simulink model "System_Model"  (Simulink 7.6)
settings: Solver=ode15s  StartTime=0.0  StopTime=50  RelTol=1e-3
undefined symbols (not defined in the file): C, DiscIntNeverNeededParam, F, G, g, H, K, L0, m, magnitude, Nu, Nx, Q, R, u0, x01, x02, x03
libraries: fl_lib x18, nesl_utility x5, simulink x3, elec_lib x1
CloseFcn:
  | rtwprivate ssgencode ModelCloseRequest System_Model1
settings Model: Creator=Fodi  LastModifiedBy=Fodi

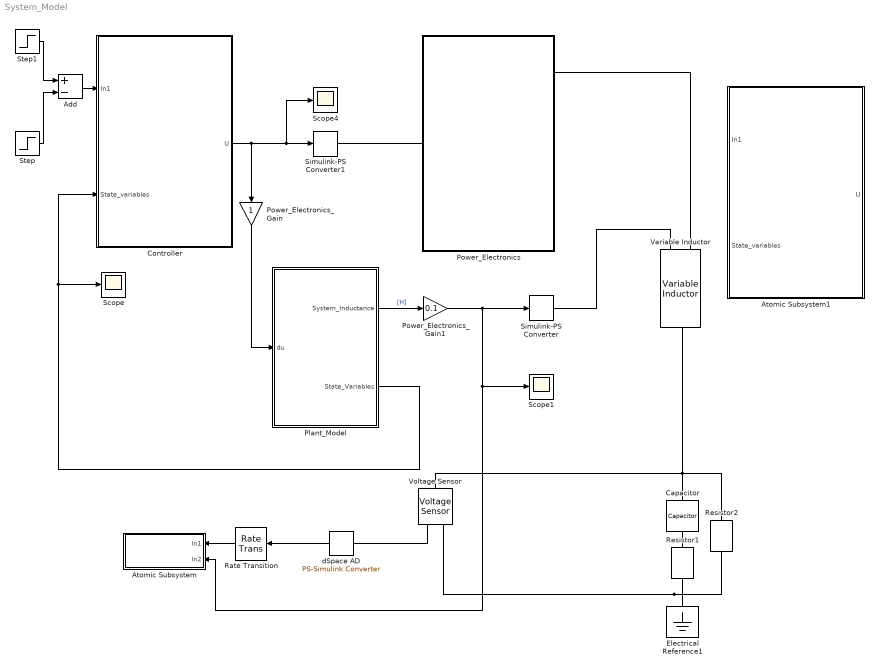
== system System_Model ==
  Add : Sum  Inputs=+-
  Atomic Subsystem : Subsystem  TreatAsAtomicUnit=on
  Atomic Subsystem1 : Subsystem  TreatAsAtomicUnit=on
  Capacitor : fl_lib/Electrical/Electrical Elements/Capacitor  DialogController=NetworkEngine.DynNeDlgSource  SystemSampleTime=-1  c=1e-6 F  v0=0 V  r=1e-6 Ohm  g=0 1/Ohm  i_Log=off  v_Log=off  vc_Log=off  LocalVarNames=|i|v|vc  LocalVarDescs=|i|v|Internal variable for voltage across capacitor term  LocalVarLogging=[0 0 0]
  Controller : Subsystem
  Electrical Reference1 : fl_lib/Electrical/Electrical Elements/Electrical Reference  DialogController=NetworkEngine.DynNeDlgSource  SystemSampleTime=-1  i_Log=off  LocalVarNames=|i  LocalVarDescs=|i  LocalVarLogging=0
  Plant_Model : Subsystem
  Power_Electronics : Subsystem
  Power_Electronics_Gain : Gain
  Power_Electronics_Gain1 : Gain  Gain=0.1
  Rate Transition : RateTransition  OutPortSampleTime=0.001
  Resistor1 : fl_lib/Electrical/Electrical Elements/Resistor  DialogController=NetworkEngine.DynNeDlgSource  SystemSampleTime=-1  R=17 Ohm  i_Log=off  v_Log=off  LocalVarNames=|i|v  LocalVarDescs=|i|v  LocalVarLogging=[0 0]
  Resistor2 : fl_lib/Electrical/Electrical Elements/Resistor  DialogController=NetworkEngine.DynNeDlgSource  SystemSampleTime=-1  R=17 Ohm  i_Log=off  v_Log=off  LocalVarNames=|i|v  LocalVarDescs=|i|v  LocalVarLogging=[0 0]
  Scope : Scope
      settings: YMin=0.00025  YMax=0.00575  SaveName=ScopeData7
  Scope1 : Scope
      settings: YMin=0.266286  YMax=0.266289  SaveName=ScopeData5
  Scope4 : Scope
      settings: YMin=0.1375  YMax=0.142  SaveName=ScopeData6
  Simulink-PS Converter : nesl_utility/Simulink-PS Converter  DialogController=NetworkEngine.DynNeUtilDlgSource  SystemSampleTime=-1  PhysicalDomain=network_engine_domain  LeftPortType=input  RightPortType=output  SubClassName=ps_input  Unit=1  AffineConversion=off  InputFilterTimeConstant=.001  UdotUserProvided=0
  Simulink-PS Converter1 : nesl_utility/Simulink-PS Converter  DialogController=NetworkEngine.DynNeUtilDlgSource  SystemSampleTime=-1  PhysicalDomain=network_engine_domain  LeftPortType=input  RightPortType=output  SubClassName=ps_input  Unit=1  AffineConversion=off  InputFilterTimeConstant=.001  UdotUserProvided=0
  Step : Step  Time=20  After=0.0003  SampleTime=0
  Step1 : Step  Time=0  After=0.001  SampleTime=0
  Variable Inductor : elec_lib/Passive Devices/Variable Inductor  DialogController=NetworkEngine.DynNeDlgSource  SystemSampleTime=-1  prm=2  Lmin=1e-6 H  g=1e-9 1/Ohm  i0=0 A  phi0=0 Wb  LocalVarLogging=[]
  Voltage Sensor : fl_lib/Electrical/Electrical Sensors/Voltage Sensor  DialogController=NetworkEngine.DynNeDlgSource  SystemSampleTime=-1  i1_Log=off  v1_Log=off  LocalVarNames=|i1|v1  LocalVarDescs=|i1|v1  LocalVarLogging=[0 0]
  dSpace AD : nesl_utility/PS-Simulink Converter  DialogController=NetworkEngine.DynNeUtilDlgSource  SystemSampleTime=-1  PhysicalDomain=network_engine_domain  LeftPortType=input  RightPortType=output  SubClassName=ps_output  Unit=1  AffineConversion=off
  wires:
  Plant_Model/1(System_Inductance) -> Power_Electronics_Gain1/1  "[H]"
  Controller/1(U) -> Power_Electronics_Gain/1, Simulink-PS Converter1/1, Scope4/1
  Power_Electronics_Gain/1 -> Plant_Model/1(du)
  Plant_Model/2(State_Variables) -> Controller/2(State_variables), Scope/1
  Power_Electronics_Gain1/1 -> Simulink-PS Converter/1, Atomic Subsystem/2(In2), Scope1/1
  Add/1 -> Controller/1(In1)
  Step1/1 -> Add/1
  Step/1 -> Add/2
  dSpace AD/1 -> Rate Transition/1
  Rate Transition/1 -> Atomic Subsystem/1(In1)
  connections:
  Simulink-PS Converter1/RConn1 -- Power_Electronics/LConn1
  Power_Electronics/RConn1 -- Variable Inductor/LConn2
  Variable Inductor/RConn1 -- Voltage Sensor/LConn1 -- Capacitor/LConn1 -- Resistor2/LConn1
  Resistor1/RConn1 -- Electrical Reference1/LConn1 -- Voltage Sensor/RConn2 -- Resistor2/RConn1
  Simulink-PS Converter/RConn1 -- Variable Inductor/LConn1
  Voltage Sensor/RConn1 -- dSpace AD/LConn1
  Capacitor/RConn1 -- Resistor1/LConn1

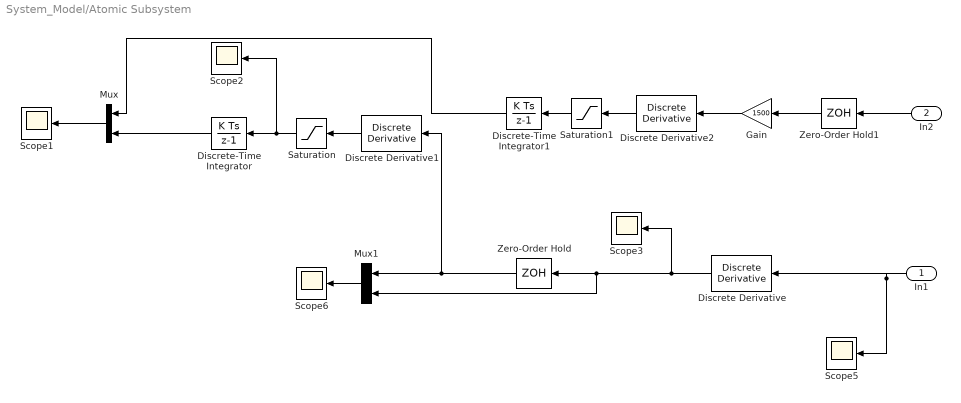
== system System_Model/Atomic Subsystem ==
  In1 : Inport
  In2 : Inport  Port=2
  Discrete Derivative : simulink/Discrete/Discrete Derivative  SystemSampleTime=-1  gainval=1.0  ICPrevScaledInput=0.0  OutMin=[]  OutMax=[]  OutDataType=fixdt(1, 16)  OutScaling=2^-10  DoSatur=off
  Discrete Derivative1 : simulink/Discrete/Discrete Derivative  SystemSampleTime=-1  gainval=1.0  ICPrevScaledInput=0.0  OutMin=[]  OutMax=[]  OutDataType=fixdt(1, 16)  OutScaling=2^-10  DoSatur=off
  Discrete Derivative2 : simulink/Discrete/Discrete Derivative  SystemSampleTime=-1  gainval=1.0  ICPrevScaledInput=0.0  OutMin=[]  OutMax=[]  OutDataType=fixdt(1, 16)  OutScaling=2^-10  DoSatur=off
  Discrete-Time Integrator : DiscreteIntegrator  SampleTime=-1  ICPrevOutput=DiscIntNeverNeededParam  ICPrevScaledInput=DiscIntNeverNeededParam
  Discrete-Time Integrator1 : DiscreteIntegrator  SampleTime=-1  ICPrevOutput=DiscIntNeverNeededParam  ICPrevScaledInput=DiscIntNeverNeededParam
  Gain : Gain  Gain=1500
  Mux : Mux  Inputs=2
  Mux1 : Mux  Inputs=2
  Saturation : Saturate  UpperLimit=10  LowerLimit=-10
  Saturation1 : Saturate  UpperLimit=10  LowerLimit=-10
  Scope{1..3,5..6} (5 alike) : Scope
      Scope1 settings: YMin=-6  YMax=-1.75  SaveName=ScopeData9
      Scope2 settings: YMin=-1.75e-008  YMax=2e-008  SaveName=ScopeData10
      Scope3 settings: YMin=-600  YMax=600  SaveName=ScopeData8
      Scope5 settings: YMin=-0.43  YMax=-0.2  SaveName=ScopeData11
      Scope6 settings: YMin=18.8348  YMax=18.8348  SaveName=ScopeData16
  Zero-Order Hold : ZeroOrderHold  SampleTime=1/20
  Zero-Order Hold1 : ZeroOrderHold  SampleTime=1/20
  wires:
  In1/1 -> Scope5/1, Discrete Derivative/1
  Zero-Order Hold/1 -> Discrete Derivative1/1, Mux1/1
  Discrete Derivative/1 -> Scope3/1, Zero-Order Hold/1, Mux1/2
  Saturation/1 -> Discrete-Time Integrator/1, Scope2/1
  Mux/1 -> Scope1/1
  Discrete-Time Integrator/1 -> Mux/2
  In2/1 -> Zero-Order Hold1/1
  Gain/1 -> Discrete Derivative2/1
  Discrete Derivative2/1 -> Saturation1/1
  Saturation1/1 -> Discrete-Time Integrator1/1
  Discrete-Time Integrator1/1 -> Mux/1
  Zero-Order Hold1/1 -> Gain/1
  Discrete Derivative1/1 -> Saturation/1
  Mux1/1 -> Scope6/1

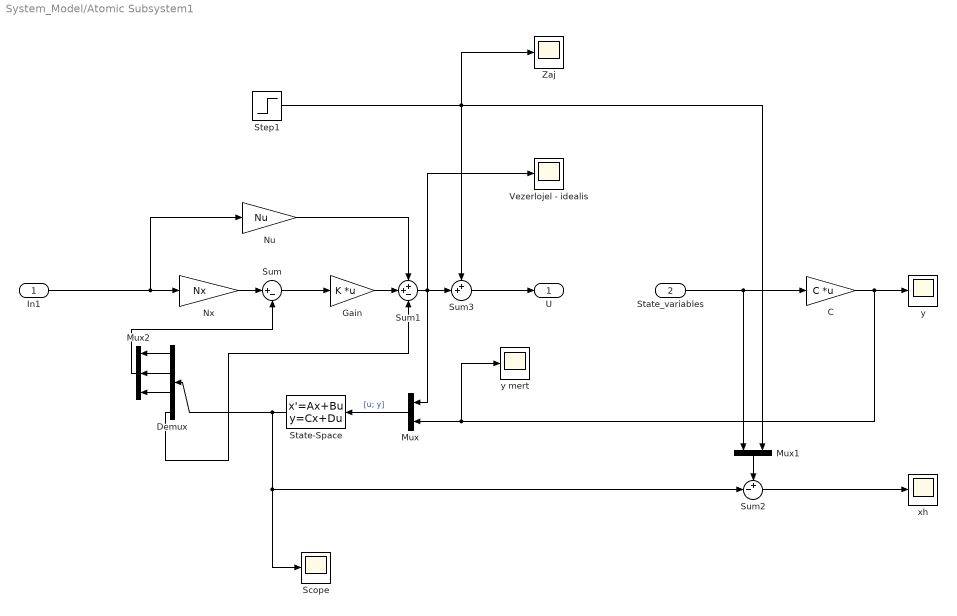
== system System_Model/Atomic Subsystem1 ==
  In1 : Inport
  State_variables : Inport  Port=2
  C : Gain  Gain=C  Multiplication=Matrix(K*u)
  Demux : Demux
  Gain : Gain  Gain=K  Multiplication=Matrix(K*u)
  Mux : Mux  Inputs=2
  Mux1 : Mux  Inputs=2
  Mux2 : Mux  Inputs=3
  Nu : Gain  Gain=Nu
  Nx : Gain  Gain=Nx
  Scope : Scope
      settings: SaveName=xb1
  State-Space : StateSpace  A=F  B=[H G]  C=eye(size(F))  D=zeros(size(F,1),size([H G],2))
  Step1 : Step  Time=2  After=0  SampleTime=0
  Sum : Sum  Inputs=|+-
  Sum1 : Sum  Inputs=++-
  Sum2 : Sum  Inputs=+-|
  Sum3 : Sum  Inputs=++|
  Vezerlojel - idealis : Scope
      settings: TimeRange=10  YMin=-1  YMax=3  SaveName=u1
  Zaj : Scope
      settings: SaveName=ScopeData12
  xh : Scope
      settings: TimeRange=10  YMin=-0.02  YMax=0.12  SaveName=ScopeData13
  y : Scope
      settings: TimeRange=10  YMin=0  YMax=0.0025  SaveName=y1
  y mert : Scope
      settings: TimeRange=5  YMin=0  YMax=0.003  SaveName=ym1
  U : Outport
  wires:
  In1/1 -> Nx/1, Nu/1
  Nx/1 -> Sum/1
  Nu/1 -> Sum1/1
  Gain/1 -> Sum1/2
  Sum/1 -> Gain/1
  Sum1/1 -> Mux/1, Sum3/2, Vezerlojel - idealis/1
  State_variables/1 -> C/1, Mux1/1
  State-Space/1 -> Demux/1, Sum2/2, Scope/1
  Mux/1 -> State-Space/1  "[u; y]"
  Step1/1 -> Sum3/1, Mux1/2, Zaj/1
  Sum3/1 -> U/1
  Mux1/1 -> Sum2/1
  Mux2/1 -> Sum/2
  Demux/4 -> Sum1/3
  Demux/1 -> Mux2/1
  Demux/2 -> Mux2/2
  Demux/3 -> Mux2/3
  Sum2/1 -> xh/1
  C/1 -> y/1, Mux/2, y mert/1

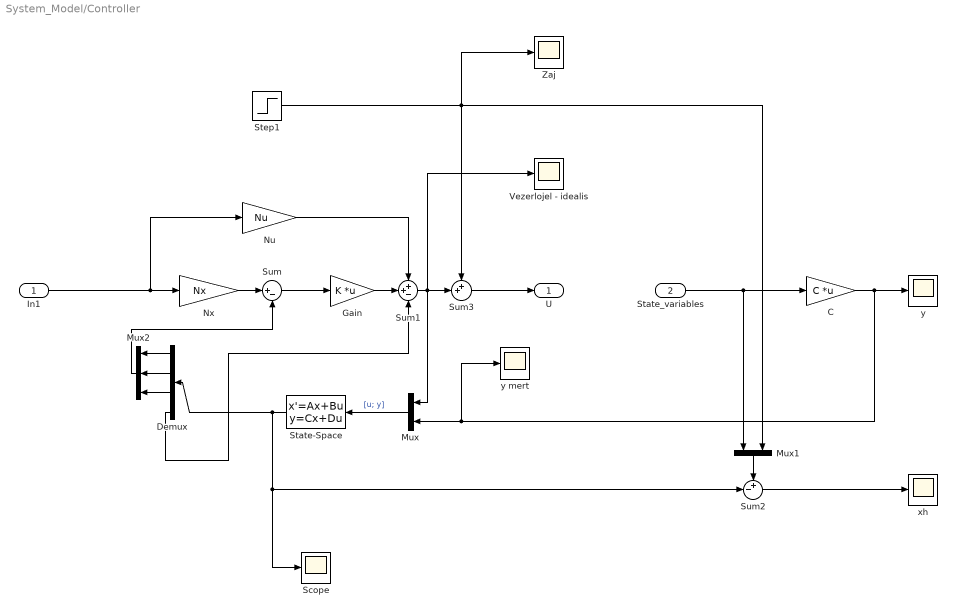
== system System_Model/Controller ==
  In1 : Inport
  State_variables : Inport  Port=2
  C : Gain  Gain=C  Multiplication=Matrix(K*u)
  Demux : Demux
  Gain : Gain  Gain=K  Multiplication=Matrix(K*u)
  Mux : Mux  Inputs=2
  Mux1 : Mux  Inputs=2
  Mux2 : Mux  Inputs=3
  Nu : Gain  Gain=Nu
  Nx : Gain  Gain=Nx
  Scope : Scope
      settings: SaveName=xb
  State-Space : StateSpace  A=F  B=[H G]  C=eye(size(F))  D=zeros(size(F,1),size([H G],2))
  Step1 : Step  Time=2  After=0  SampleTime=0
  Sum : Sum  Inputs=|+-
  Sum1 : Sum  Inputs=++-
  Sum2 : Sum  Inputs=+-|
  Sum3 : Sum  Inputs=++|
  Vezerlojel - idealis : Scope
      settings: TimeRange=10  YMin=-1  YMax=3  SaveName=u
  Zaj : Scope
      settings: SaveName=ScopeData2
  xh : Scope
      settings: TimeRange=10  YMin=-0.02  YMax=0.12  SaveName=ScopeData4
  y : Scope
      settings: TimeRange=10  YMin=0  YMax=0.0025  SaveName=y
  y mert : Scope
      settings: TimeRange=5  YMin=0  YMax=0.003  SaveName=ym
  U : Outport
  wires:
  In1/1 -> Nx/1, Nu/1
  Nx/1 -> Sum/1
  Nu/1 -> Sum1/1
  Gain/1 -> Sum1/2
  Sum/1 -> Gain/1
  Sum1/1 -> Mux/1, Sum3/2, Vezerlojel - idealis/1
  State_variables/1 -> C/1, Mux1/1
  State-Space/1 -> Demux/1, Sum2/2, Scope/1
  Mux/1 -> State-Space/1  "[u; y]"
  Step1/1 -> Sum3/1, Mux1/2, Zaj/1
  Sum3/1 -> U/1
  Mux1/1 -> Sum2/1
  Mux2/1 -> Sum/2
  Demux/4 -> Sum1/3
  Demux/1 -> Mux2/1
  Demux/2 -> Mux2/2
  Demux/3 -> Mux2/3
  Sum2/1 -> xh/1
  C/1 -> y/1, Mux/2, y mert/1

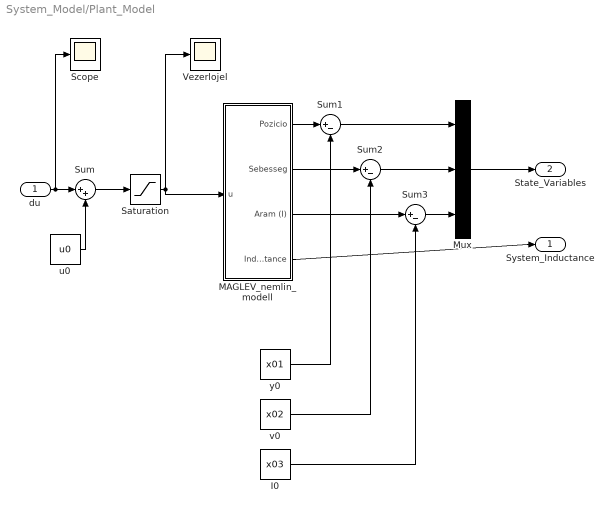
== system System_Model/Plant_Model ==
  du : Inport
  I0 : Constant  Value=x03
  MAGLEV_nemlin_modell : Subsystem
  Mux : Mux  Inputs=3
  Saturation : Saturate  UpperLimit=30  LowerLimit=-30
  Scope : Scope
  Sum : Sum  Inputs=|++
  Sum1 : Sum  Inputs=|+-
  Sum2 : Sum  Inputs=|+-
  Sum3 : Sum  Inputs=|+-
  Vezerlojel : Scope
      settings: TimeRange=10  YMin=11  YMax=16
  u0 : Constant  Value=u0
  v0 : Constant  Value=x02
  y0 : Constant  Value=x01
  System_Inductance : Outport
  State_Variables : Outport  Port=2
  wires:
  y0/1 -> Sum1/2
  v0/1 -> Sum2/2
  I0/1 -> Sum3/2
  MAGLEV_nemlin_modell/3(Aram (I)) -> Sum3/1
  Sum3/1 -> Mux/3
  Sum2/1 -> Mux/2
  Sum1/1 -> Mux/1
  u0/1 -> Sum/2
  Mux/1 -> State_Variables/1
  MAGLEV_nemlin_modell/2(Sebesseg) -> Sum2/1
  MAGLEV_nemlin_modell/1(Pozicio) -> Sum1/1
  du/1 -> Scope/1, Sum/1
  Sum/1 -> Saturation/1
  Saturation/1 -> MAGLEV_nemlin_modell/1(u), Vezerlojel/1
  MAGLEV_nemlin_modell/4(Inductance) -> System_Inductance/1

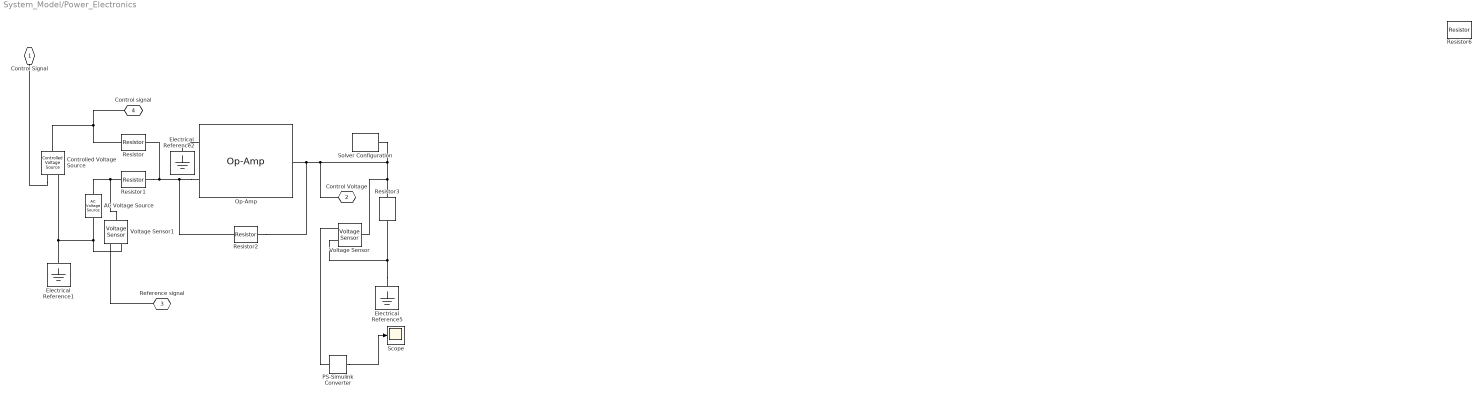
== system System_Model/Power_Electronics ==
  AC Voltage Source : fl_lib/Electrical/Electrical Sources/AC Voltage Source  DialogController=NetworkEngine.DynNeDlgSource  SystemSampleTime=-1  amp=10 V  shift=0 rad  omega=20 Hz  i_Log=off  v_Log=off  LocalVarNames=|i|v  LocalVarDescs=|i|v  LocalVarLogging=[0 0]
  Controlled Voltage Source : fl_lib/Electrical/Electrical Sources/Controlled Voltage Source  DialogController=NetworkEngine.DynNeDlgSource  SystemSampleTime=-1  i_Log=off  v_Log=off  LocalVarNames=|i|v  LocalVarDescs=|i|v  LocalVarLogging=[0 0]
  Electrical Reference1 : fl_lib/Electrical/Electrical Elements/Electrical Reference  DialogController=NetworkEngine.DynNeDlgSource  SystemSampleTime=-1  i_Log=off  LocalVarNames=|i  LocalVarDescs=|i  LocalVarLogging=0
  Electrical Reference2 : fl_lib/Electrical/Electrical Elements/Electrical Reference  DialogController=NetworkEngine.DynNeDlgSource  SystemSampleTime=-1  i_Log=off  LocalVarNames=|i  LocalVarDescs=|i  LocalVarLogging=0
  Electrical Reference5 : fl_lib/Electrical/Electrical Elements/Electrical Reference  DialogController=NetworkEngine.DynNeDlgSource  SystemSampleTime=-1  i_Log=off  LocalVarNames=|i  LocalVarDescs=|i  LocalVarLogging=0
  Op-Amp : fl_lib/Electrical/Electrical Elements/Op-Amp  DialogController=NetworkEngine.DynNeDlgSource  SystemSampleTime=-1  i1_Log=off  v1_Log=off  outI_Log=off  LocalVarNames=|i1|v1|outI  LocalVarDescs=|i1|v1|outI  LocalVarLogging=[0 0 0]
  PS-Simulink Converter : nesl_utility/PS-Simulink Converter  DialogController=NetworkEngine.DynNeUtilDlgSource  SystemSampleTime=-1  PhysicalDomain=network_engine_domain  LeftPortType=input  RightPortType=output  SubClassName=ps_output  Unit=1  AffineConversion=off
  Resistor{,1..2,6} (4 alike) : fl_lib/Electrical/Electrical Elements/Resistor  DialogController=NetworkEngine.DynNeDlgSource  SystemSampleTime=-1  R=1 kOhm  i_Log=off  v_Log=off  LocalVarNames=|i|v  LocalVarDescs=|i|v  LocalVarLogging=[0 0]
  Resistor3 : fl_lib/Electrical/Electrical Elements/Resistor  DialogController=NetworkEngine.DynNeDlgSource  SystemSampleTime=-1  R=100 kOhm  i_Log=off  v_Log=off  LocalVarNames=|i|v  LocalVarDescs=|i|v  LocalVarLogging=[0 0]
  Scope : Scope
      settings: SaveName=ScopeData3
  Solver Configuration : nesl_utility/Solver Configuration  DialogController=NetworkEngine.DynNeUtilDlgSource  SystemSampleTime=-1  PhysicalDomain=network_engine_domain  LeftPortType=input  RightPortType=generic  SubClassName=solver  Accelerate=off  Profile=off  ResidualTolerance=1e-9  MaxNonlinIter=3  MaxModeIter=2  DoFixedCost=off  UseLocalSampling=off  DoDC=off  LinearAlgebra=Sparse  LocalSolverSampleTime=.001  LocalSolverChoice=NE_BACKWARD_EULER_ADVANCER  UseLocalSolver=off
  Voltage Sensor : fl_lib/Electrical/Electrical Sensors/Voltage Sensor  DialogController=NetworkEngine.DynNeDlgSource  SystemSampleTime=-1  i1_Log=off  v1_Log=off  LocalVarNames=|i1|v1  LocalVarDescs=|i1|v1  LocalVarLogging=[0 0]
  Voltage Sensor1 : fl_lib/Electrical/Electrical Sensors/Voltage Sensor  DialogController=NetworkEngine.DynNeDlgSource  SystemSampleTime=-1  i1_Log=off  v1_Log=off  LocalVarNames=|i1|v1  LocalVarDescs=|i1|v1  LocalVarLogging=[0 0]
  Control Signal : PMIOPort  Tag=PMCPort  Port=1  Side=Left
  Control Voltage : PMIOPort  Tag=PMCPort  Port=2  Side=Right
  Reference signal : PMIOPort  Tag=PMCPort  Port=3  Side=Right
  Control signal : PMIOPort  Tag=PMCPort  Port=4  Side=Right
  wires:
  PS-Simulink Converter/1 -> Scope/1
  connections:
  Op-Amp/LConn2 -- Resistor2/LConn1 -- Resistor/RConn1 -- Resistor1/RConn1
  Solver Configuration/RConn1 -- Resistor3/LConn1 -- Voltage Sensor/LConn1 -- Control Voltage/RConn1 -- Op-Amp/RConn1 -- Resistor2/RConn1
  Electrical Reference5/LConn1 -- Voltage Sensor/RConn2 -- Resistor3/RConn1
  Controlled Voltage Source/LConn1 -- Resistor/LConn1 -- Control signal/RConn1
  AC Voltage Source/RConn1 -- Voltage Sensor1/RConn2 -- Controlled Voltage Source/RConn2 -- Electrical Reference1/LConn1
  AC Voltage Source/LConn1 -- Resistor1/LConn1 -- Voltage Sensor1/LConn1
  Op-Amp/LConn1 -- Electrical Reference2/LConn1
  Voltage Sensor/RConn1 -- PS-Simulink Converter/LConn1
  Controlled Voltage Source/RConn1 -- Control Signal/RConn1
  Voltage Sensor1/RConn1 -- Reference signal/RConn1

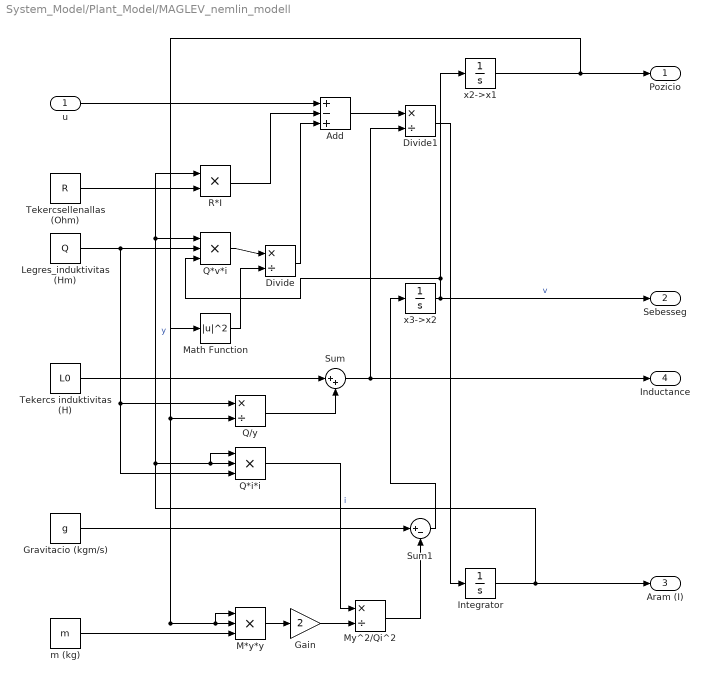
== system System_Model/Plant_Model/MAGLEV_nemlin_modell ==
  u : Inport  Tag=v
  Add : Sum  Inputs=+-+
  Divide : Product  Inputs=*/
  Divide1 : Product  Inputs=*/
  Gain : Gain  Gain=2
  Gravitacio (kgm/s) : Constant  Value=g
  Integrator : Integrator  InitialCondition=x03
  Legres_induktivitas (Hm) : Constant  Value=Q
  M*y*y : Product  Inputs=3  RndMeth=Zero
  Math Function : Math  Operator=magnitude^2  SaturateOnIntegerOverflow=on
  My^2/Qi^2 : Product  Inputs=*/
  Q*i*i : Product  Inputs=3  RndMeth=Zero
  Q*v*i : Product  Inputs=3  RndMeth=Zero
  Q/y : Product  Inputs=*/
  R*I : Product  RndMeth=Zero
  Sum : Sum  Inputs=|++
  Sum1 : Sum  Inputs=|+-
  Tekercs induktivitas (H) : Constant  Value=L0
  Tekercsellenallas (Ohm) : Constant  Value=R
  m (kg) : Constant  Value=m
  x2->x1 : Integrator  InitialCondition=x01
  x3->x2 : Integrator  InitialCondition=0.01
  Pozicio : Outport
  Sebesseg : Outport  Port=2
  Aram (I) : Outport  Port=3
  Inductance : Outport  Port=4
  wires:
  x2->x1/1 -> Pozicio/1, Q/y/2, Math Function/1, M*y*y/2, M*y*y/1  "y"
  Sum1/1 -> x3->x2/1
  Gravitacio (kgm/s)/1 -> Sum1/1
  My^2/Qi^2/1 -> Sum1/2
  Gain/1 -> My^2/Qi^2/2
  M*y*y/1 -> Gain/1
  Sum/1 -> Divide1/2, Inductance/1
  Tekercs induktivitas (H)/1 -> Sum/1
  Q/y/1 -> Sum/2
  Math Function/1 -> Divide/2
  Divide/1 -> Add/3
  Q*v*i/1 -> Divide/1
  R*I/1 -> Add/2
  Divide1/1 -> Integrator/1
  Add/1 -> Divide1/1
  u/1 -> Add/1
  m (kg)/1 -> M*y*y/3
  Legres_induktivitas (Hm)/1 -> Q*v*i/2, Q/y/1, Q*i*i/3
  Tekercsellenallas (Ohm)/1 -> R*I/2
  Q*i*i/1 -> My^2/Qi^2/1
  x3->x2/1 -> Q*v*i/3, x2->x1/1, Sebesseg/1  "v"
  Integrator/1 -> Aram (I)/1, Q*i*i/2, Q*i*i/1, Q*v*i/1, R*I/1  "i"
